simulink model "Hierarchy1_tmp"  (Simulink 8.3)
settings: Solver=ode45  StartTime=0.0  StopTime=10.0  RelTol=1e-3
settings Model: Creator=scaife  LastModifiedBy=bourbouh  CovSFcnEnable=on  ExtModeAutoUpdateStatusClock=off
settings DataIOCC: SignalLoggingName=sigsOut
settings DebuggingCC: SaveWithParameterizedLinksMsg=none  SignalResolutionControl=TryResolveAllWithWarning  SolverPrmCheckMsg=none  MultiTaskDSMMsg=warning  MultiTaskCondExecSysMsg=none  FrameProcessingCompatibilityMsg=error  StateNameClashWarn=none  StrictBusMsg=None
settings HardwareCC: TargetUnknown=on
settings SFSimCC: SimParseCustomCode=off
settings GRTTargetCC: GeneratePreprocessorConditionals=Use local settings

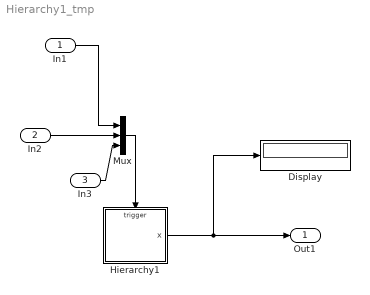
== system Hierarchy1_tmp ==
  In1 : Inport
  In2 : Inport  Port=2
  In3 : Inport  Port=3
  Display : Display
  Hierarchy1 : Stateflow chart  TreatAsAtomicUnit=on
      settings: PermitHierarchicalResolution=ParametersOnly
  Mux : Mux  Inputs=3
  Out1 : Outport
  wires:
  Hierarchy1/1(x) -> Out1/1, Display/1
  Mux/1 -> Hierarchy1/Trigger
  In1/1 -> Mux/1
  In2/1 -> Mux/2
  In3/1 -> Mux/3

== stateflow chart Hierarchy1 ==
  state TOP/ en:x+=1000000; ex:x=0;
    state N1/
      en:x+=10000;
      ex:x-=10000;
      state A/
        en: x+=10;
      state B/
        en: x-=10;
      (default) -> A
      A -> B : S{x+=1;}
      B -> A : R{x-=1;}
    state N2/
      en:x+=100000;
      ex:x-=100000;
      state C/
        en: x+=1000;
      state D/
        en: x-=1000;
      (default) -> C
      C -> D : S{x+=100;}
      D -> C : R{x-=100;}
    N2 -> N1 : T
    (default) -> N1
    N1 -> N2 : T
  (default) -> TOP/ en:x+=1000000; ex:x=0;
  data: x output double
  events: S input EITHER_EDGE_EVENT; R input EITHER_EDGE_EVENT; T input EITHER_EDGE_EVENT
